simulink library "inp"  (R2021b)
settings: Solver=VariableStepAuto  StartTime=0.0  StopTime=10.0  RelTol=1e-3
undefined symbols (not defined in the file): C_TASK_5MS_S, FALSE, KINP_AcoreReadyToSlp_flg_ovrdflg, KINP_AcoreReadyToSlp_flg_ovrdval, KINP_AllowMovThd_OTA_enum_ovrdflg, KINP_AllowMovThd_OTA_enum_ovrdval, KINP_APSAngleTarget_Deg_ovrdflg, KINP_APSAngleTarget_Deg_ovrdval, KINP_APSDecReq_mps2_ovrdflg, KINP_APSDecReq_mps2_ovrdval, KINP_APSDecReqA_flg_ovrdflg, KINP_APSDecReqA_flg_ovrdval, KINP_APSDFLL_cm_ovrdflg, KINP_APSDFLL_cm_ovrdval, KINP_APSDFLR_cm_ovrdflg, KINP_APSDFLR_cm_ovrdval, KINP_APSDRLL_cm_ovrdflg, KINP_APSDRLL_cm_ovrdval, KINP_APSDRLR_cm_ovrdflg, KINP_APSDRLR_cm_ovrdval, KINP_APSExitCondition_enum_ovrdflg, KINP_APSExitCondition_enum_ovrdval, KINP_APSHWVer_enum_ovrdflg, KINP_APSHWVer_enum_ovrdval, KINP_APSProgressPCT_pct_ovrdflg, KINP_APSProgressPCT_pct_ovrdval, KINP_APSReq_enum_ovrdflg, KINP_APSReq_enum_ovrdval, KINP_APSRQDisplay_enum_ovrdflg, KINP_APSRQDisplay_enum_ovrdval, KINP_APSRqEPASCtrl_flg_ovrdflg, KINP_APSRqEPASCtrl_flg_ovrdval, KINP_APSShiftPosnReq_enum_ovrdval, KINP_APSShiftPosnReq_enum_ovrflg, KINP_APSSpeedCMD_kph_ovrdval, KINP_APSSpeedCMD_kph_ovrflg, KINP_APSStaSystem_enum_ovrdflg, KINP_APSStaSystem_enum_ovrdval, KINP_APSSWVer_enum_ovrdflg, KINP_APSSWVer_enum_ovrdval, KINP_APSVMCReqA_flg_ovrdval, KINP_APSVMCReqA_flg_ovrflg, KINP_APSVRqEPASCtrl_flg_ovrdflg, KINP_APSVRqEPASCtrl_flg_ovrdval, KINP_AuxBattVolmV_mV_ovrdflg, KINP_AuxBattVolmV_mV_ovrdval, KINP_CAASSta_enum_ovrdflg, KINP_CAASSta_enum_ovrdval, KINP_CAASVMCReqA_flg_ovrdval, KINP_CAASVMCReqA_flg_ovrflg, KINP_Chime_enum_ovrdflg, KINP_Chime_enum_ovrdval, KINP_ClearDTCcmd_flg_ovrdflg, KINP_ClearDTCcmd_flg_ovrdval, KINP_EvccAplusPwrUpReq_flg_ovrdflg, KINP_EvccAplusPwrUpReq_flg_ovrdval, KINP_LFID_raw_ovrdval, KINP_LFID_raw_ovrflg, KINP_LRID_raw_ovrdval, KINP_MemOffsetAccX_raw16_ovrdflg ... (+118)
libraries: FVT_lib x595, hcu_lib x1
(part 12 of 27)

== system inp/INP/CAN1/SignalCheck/FCM3 ==
  BHAL_outputs : Inport
  inp_CanValid_bus : Inport  Port=2
  ACCObjDist : FVT_lib/inp/can_signal_template  SystemSampleTime=-1  VariantActivationTime=update diagram  Latency=0  AutoFrameSizeCalculation=off
      link override defval: Value=KINP_ACCObjDist_m_defval
      link override fftdec: Value=KINP_ACCObjDist_m_fftdec
      link override fftinc: Value=KINP_ACCObjDist_m_fftinc
      link override fftlim: Value=KINP_ACCObjDist_m_fftlim
      link override invalid: Value=KINP_ACCObjDist_m_invalid
      link override ovrdflg: Value=KINP_ACCObjDist_m_ovrdflg
      link override ovrdval: Value=KINP_ACCObjDist_m_ovrdval
      link override setvalid: Value=KINP_ACCObjDist_m_setvalid
      link override srvcflg: Value=KINP_ACCObjDist_m_srvcflg
      link override srvcval: Value=KINP_ACCObjDist_m_srvcval
  ACCObjRelSpd : FVT_lib/inp/can_signal_template  SystemSampleTime=-1  VariantActivationTime=update diagram  Latency=0  AutoFrameSizeCalculation=off
      link override defval: Value=KINP_ACCObjRelSpd_mps_defval
      link override fftdec: Value=KINP_ACCObjRelSpd_mps_fftdec
      link override fftinc: Value=KINP_ACCObjRelSpd_mps_fftinc
      link override fftlim: Value=KINP_ACCObjRelSpd_mps_fftlim
      link override invalid: Value=KINP_ACCObjRelSpd_mps_invalid
      link override ovrdflg: Value=KINP_ACCObjRelSpd_mps_ovrdflg
      link override ovrdval: Value=KINP_ACCObjRelSpd_mps_ovrdval
      link override setvalid: Value=KINP_ACCObjRelSpd_mps_setvalid
      link override srvcflg: Value=KINP_ACCObjRelSpd_mps_srvcflg
      link override srvcval: Value=KINP_ACCObjRelSpd_mps_srvcval
  ADASForceIdle : FVT_lib/inp/can_signal_template  SystemSampleTime=-1  VariantActivationTime=update diagram  Latency=0  AutoFrameSizeCalculation=off
      link override defval: Value=KINP_ADASForceIdle_flg_defval
      link override fftdec: Value=KINP_ADASForceIdle_flg_fftdec
      link override fftinc: Value=KINP_ADASForceIdle_flg_fftinc
      link override fftlim: Value=KINP_ADASForceIdle_flg_fftlim
      link override invalid: Value=KINP_ADASForceIdle_flg_invalid
      link override ovrdflg: Value=KINP_ADASForceIdle_flg_ovrdflg
      link override ovrdval: Value=KINP_ADASForceIdle_flg_ovrdval
      link override setvalid: Value=KINP_ADASForceIdle_flg_setvalid
      link override srvcflg: Value=KINP_ADASForceIdle_flg_srvcflg
      link override srvcval: Value=KINP_ADASForceIdle_flg_srvcval
  FCM3CSErr : FVT_lib/inp/can_signal_template  SystemSampleTime=-1  VariantActivationTime=update diagram  Latency=0  AutoFrameSizeCalculation=off
      link override defval: Value=KINP_FCM3CSErr_flg_defval
      link override fftdec: Value=KINP_FCM3CSErr_flg_fftdec
      link override fftinc: Value=KINP_FCM3CSErr_flg_fftinc
      link override fftlim: Value=KINP_FCM3CSErr_flg_fftlim
      link override invalid: Value=KINP_FCM3CSErr_flg_invalid
      link override ovrdflg: Value=KINP_FCM3CSErr_flg_ovrdflg
      link override ovrdval: Value=KINP_FCM3CSErr_flg_ovrdval
      link override setvalid: Value=KINP_FCM3CSErr_flg_setvalid
      link override srvcflg: Value=KINP_FCM3CSErr_flg_srvcflg
      link override srvcval: Value=KINP_FCM3CSErr_flg_srvcval
  FCM3Checksum : FVT_lib/inp/can_signal_template  SystemSampleTime=-1  VariantActivationTime=update diagram  Latency=0  AutoFrameSizeCalculation=off
      link override defval: Value=KINP_FCM3Checksum_enum_defval
      link override fftdec: Value=KINP_FCM3Checksum_enum_fftdec
      link override fftinc: Value=KINP_FCM3Checksum_enum_fftinc
      link override fftlim: Value=KINP_FCM3Checksum_enum_fftlim
      link override invalid: Value=KINP_FCM3Checksum_enum_invalid
      link override ovrdflg: Value=KINP_FCM3Checksum_enum_ovrdflg
      link override ovrdval: Value=KINP_FCM3Checksum_enum_ovrdval
      link override setvalid: Value=KINP_FCM3Checksum_enum_setvalid
      link override srvcflg: Value=KINP_FCM3Checksum_enum_srvcflg
      link override srvcval: Value=KINP_FCM3Checksum_enum_srvcval
  FCM3LifeCount : FVT_lib/inp/can_signal_template  SystemSampleTime=-1  VariantActivationTime=update diagram  Latency=0  AutoFrameSizeCalculation=off
      link override defval: Value=KINP_FCM3LifeCount_enum_defval
      link override fftdec: Value=KINP_FCM3LifeCount_enum_fftdec
      link override fftinc: Value=KINP_FCM3LifeCount_enum_fftinc
      link override fftlim: Value=KINP_FCM3LifeCount_enum_fftlim
      link override invalid: Value=KINP_FCM3LifeCount_enum_invalid
      link override ovrdflg: Value=KINP_FCM3LifeCount_enum_ovrdflg
      link override ovrdval: Value=KINP_FCM3LifeCount_enum_ovrdval
      link override setvalid: Value=KINP_FCM3LifeCount_enum_setvalid
      link override srvcflg: Value=KINP_FCM3LifeCount_enum_srvcflg
      link override srvcval: Value=KINP_FCM3LifeCount_enum_srvcval
  FCM3RCErr : FVT_lib/inp/can_signal_template  SystemSampleTime=-1  VariantActivationTime=update diagram  Latency=0  AutoFrameSizeCalculation=off
      link override defval: Value=KINP_FCM3RCErr_flg_defval
      link override fftdec: Value=KINP_FCM3RCErr_flg_fftdec
      link override fftinc: Value=KINP_FCM3RCErr_flg_fftinc
      link override fftlim: Value=KINP_FCM3RCErr_flg_fftlim
      link override invalid: Value=KINP_FCM3RCErr_flg_invalid
      link override ovrdflg: Value=KINP_FCM3RCErr_flg_ovrdflg
      link override ovrdval: Value=KINP_FCM3RCErr_flg_ovrdval
      link override setvalid: Value=KINP_FCM3RCErr_flg_setvalid
      link override srvcflg: Value=KINP_FCM3RCErr_flg_srvcflg
      link override srvcval: Value=KINP_FCM3RCErr_flg_srvcval
  Terminator_{1..7} (7 alike) : Terminator
  True_VHAL_ACCObjDist_m : Constant  Value=TRUE  OutDataTypeStr=boolean
  True_VHAL_ACCObjRelSpd_mps : Constant  Value=TRUE  OutDataTypeStr=boolean
  True_VHAL_ADASForceIdle_flg : Constant  Value=TRUE  OutDataTypeStr=boolean
  True_VHAL_FCM3CSErr_flg : Constant  Value=TRUE  OutDataTypeStr=boolean
  True_VHAL_FCM3Checksum_enum : Constant  Value=TRUE  OutDataTypeStr=boolean
  True_VHAL_FCM3LifeCount_enum : Constant  Value=TRUE  OutDataTypeStr=boolean
  True_VHAL_FCM3RCErr_flg : Constant  Value=TRUE  OutDataTypeStr=boolean
  slr1_{1..7} (7 alike) : BusSelector  OutputSignals=VINP_CANMsgValidFCM3_flg
  slr_VHAL_ACCObjDist_m : BusSelector  OutputSignals=VHAL_ACCObjDist_m
  slr_VHAL_ACCObjRelSpd_mps : BusSelector  OutputSignals=VHAL_ACCObjRelSpd_mps
  slr_VHAL_ADASForceIdle_flg : BusSelector  OutputSignals=VHAL_ADASForceIdle_flg
  slr_VHAL_FCM3CSErr_flg : BusSelector  OutputSignals=VHAL_FCM3CSErr_flg
  slr_VHAL_FCM3Checksum_enum : BusSelector  OutputSignals=VHAL_FCM3Checksum_enum
  slr_VHAL_FCM3LifeCount_enum : BusSelector  OutputSignals=VHAL_FCM3LifeCount_enum
  slr_VHAL_FCM3RCErr_flg : BusSelector  OutputSignals=VHAL_FCM3RCErr_flg
  VINP_FCM3CSErr_flg : Outport
  VINP_FCM3RCErr_flg : Outport  Port=2
  VINP_ACCObjDist_m : Outport  Port=3
  VINP_ACCObjRelSpd_mps : Outport  Port=4
  VINP_ADASForceIdle_flg : Outport  Port=5
  VINP_FCM3Checksum_enum : Outport  Port=6
  VINP_FCM3LifeCount_enum : Outport  Port=7
  wires:
  BHAL_outputs/1 -> [BHAL_outputs]
  inp_CanValid_bus/1 -> [inp_CanValid_bus]
  [BHAL_outputs] -> slr_VHAL_FCM3CSErr_flg/1
  slr_VHAL_FCM3CSErr_flg/1 -> FCM3CSErr/1  "<VHAL_FCM3CSErr_flg>"
  True_VHAL_FCM3CSErr_flg/1 -> FCM3CSErr/2
  [inp_CanValid_bus] -> slr1_1/1
  slr1_1/1 -> FCM3CSErr/3  "<VINP_CANMsgValidFCM3_flg>"
  FCM3CSErr/1 -> VINP_FCM3CSErr_flg/1  "VINP_FCM3CSErr_flg"
  FCM3CSErr/2 -> Terminator_1/1
  [BHAL_outputs] -> slr_VHAL_FCM3RCErr_flg/1
  slr_VHAL_FCM3RCErr_flg/1 -> FCM3RCErr/1  "<VHAL_FCM3RCErr_flg>"
  True_VHAL_FCM3RCErr_flg/1 -> FCM3RCErr/2
  [inp_CanValid_bus] -> slr1_2/1
  slr1_2/1 -> FCM3RCErr/3  "<VINP_CANMsgValidFCM3_flg>"
  FCM3RCErr/1 -> VINP_FCM3RCErr_flg/1  "VINP_FCM3RCErr_flg"
  FCM3RCErr/2 -> Terminator_2/1
  [BHAL_outputs] -> slr_VHAL_ACCObjDist_m/1
  slr_VHAL_ACCObjDist_m/1 -> ACCObjDist/1  "<VHAL_ACCObjDist_m>"
  True_VHAL_ACCObjDist_m/1 -> ACCObjDist/2
  [inp_CanValid_bus] -> slr1_3/1
  slr1_3/1 -> ACCObjDist/3  "<VINP_CANMsgValidFCM3_flg>"
  ACCObjDist/1 -> VINP_ACCObjDist_m/1  "VINP_ACCObjDist_m"
  ACCObjDist/2 -> Terminator_3/1
  [BHAL_outputs] -> slr_VHAL_ACCObjRelSpd_mps/1
  slr_VHAL_ACCObjRelSpd_mps/1 -> ACCObjRelSpd/1  "<VHAL_ACCObjRelSpd_mps>"
  True_VHAL_ACCObjRelSpd_mps/1 -> ACCObjRelSpd/2
  [inp_CanValid_bus] -> slr1_4/1
  slr1_4/1 -> ACCObjRelSpd/3  "<VINP_CANMsgValidFCM3_flg>"
  ACCObjRelSpd/1 -> VINP_ACCObjRelSpd_mps/1  "VINP_ACCObjRelSpd_mps"
  ACCObjRelSpd/2 -> Terminator_4/1
  [BHAL_outputs] -> slr_VHAL_ADASForceIdle_flg/1
  slr_VHAL_ADASForceIdle_flg/1 -> ADASForceIdle/1  "<VHAL_ADASForceIdle_flg>"
  True_VHAL_ADASForceIdle_flg/1 -> ADASForceIdle/2
  [inp_CanValid_bus] -> slr1_5/1
  slr1_5/1 -> ADASForceIdle/3  "<VINP_CANMsgValidFCM3_flg>"
  ADASForceIdle/1 -> VINP_ADASForceIdle_flg/1  "VINP_ADASForceIdle_flg"
  ADASForceIdle/2 -> Terminator_5/1
  [BHAL_outputs] -> slr_VHAL_FCM3Checksum_enum/1
  slr_VHAL_FCM3Checksum_enum/1 -> FCM3Checksum/1  "<VHAL_FCM3Checksum_enum>"
  True_VHAL_FCM3Checksum_enum/1 -> FCM3Checksum/2
  [inp_CanValid_bus] -> slr1_6/1
  slr1_6/1 -> FCM3Checksum/3  "<VINP_CANMsgValidFCM3_flg>"
  FCM3Checksum/1 -> VINP_FCM3Checksum_enum/1  "VINP_FCM3Checksum_enum"
  FCM3Checksum/2 -> Terminator_6/1
  [BHAL_outputs] -> slr_VHAL_FCM3LifeCount_enum/1
  slr_VHAL_FCM3LifeCount_enum/1 -> FCM3LifeCount/1  "<VHAL_FCM3LifeCount_enum>"
  True_VHAL_FCM3LifeCount_enum/1 -> FCM3LifeCount/2
  [inp_CanValid_bus] -> slr1_7/1
  slr1_7/1 -> FCM3LifeCount/3  "<VINP_CANMsgValidFCM3_flg>"
  FCM3LifeCount/1 -> VINP_FCM3LifeCount_enum/1  "VINP_FCM3LifeCount_enum"
  FCM3LifeCount/2 -> Terminator_7/1

== system inp/INP/CAN1/SignalCheck/FCM4 ==
  BHAL_outputs : Inport
  inp_CanValid_bus : Inport  Port=2
  ACCSetSpeed : FVT_lib/inp/can_signal_template  SystemSampleTime=-1  VariantActivationTime=update diagram  Latency=0  AutoFrameSizeCalculation=off
      link override defval: Value=KINP_ACCSetSpeed_enum_defval
      link override fftdec: Value=KINP_ACCSetSpeed_enum_fftdec
      link override fftinc: Value=KINP_ACCSetSpeed_enum_fftinc
      link override fftlim: Value=KINP_ACCSetSpeed_enum_fftlim
      link override invalid: Value=KINP_ACCSetSpeed_enum_invalid
      link override ovrdflg: Value=KINP_ACCSetSpeed_enum_ovrdflg
      link override ovrdval: Value=KINP_ACCSetSpeed_enum_ovrdval
      link override setvalid: Value=KINP_ACCSetSpeed_enum_setvalid
      link override srvcflg: Value=KINP_ACCSetSpeed_enum_srvcflg
      link override srvcval: Value=KINP_ACCSetSpeed_enum_srvcval
  ACCSetSpeedDisp : FVT_lib/inp/can_signal_template  SystemSampleTime=-1  VariantActivationTime=update diagram  Latency=0  AutoFrameSizeCalculation=off
      link override defval: Value=KINP_ACCSetSpeedDisp_enum_defval
      link override fftdec: Value=KINP_ACCSetSpeedDisp_enum_fftdec
      link override fftinc: Value=KINP_ACCSetSpeedDisp_enum_fftinc
      link override fftlim: Value=KINP_ACCSetSpeedDisp_enum_fftlim
      link override invalid: Value=KINP_ACCSetSpeedDisp_enum_invalid
      link override ovrdflg: Value=KINP_ACCSetSpeedDisp_enum_ovrdflg
      link override ovrdval: Value=KINP_ACCSetSpeedDisp_enum_ovrdval
      link override setvalid: Value=KINP_ACCSetSpeedDisp_enum_setvalid
      link override srvcflg: Value=KINP_ACCSetSpeedDisp_enum_srvcflg
      link override srvcval: Value=KINP_ACCSetSpeedDisp_enum_srvcval
  ADASACCSta : FVT_lib/inp/can_signal_template  SystemSampleTime=-1  VariantActivationTime=update diagram  Latency=0  AutoFrameSizeCalculation=off
      link override defval: Value=KINP_ADASACCSta_enum_defval
      link override fftdec: Value=KINP_ADASACCSta_enum_fftdec
      link override fftinc: Value=KINP_ADASACCSta_enum_fftinc
      link override fftlim: Value=KINP_ADASACCSta_enum_fftlim
      link override invalid: Value=KINP_ADASACCSta_enum_invalid
      link override ovrdflg: Value=KINP_ADASACCSta_enum_ovrdflg
      link override ovrdval: Value=KINP_ADASACCSta_enum_ovrdval
      link override setvalid: Value=KINP_ADASACCSta_enum_setvalid
      link override srvcflg: Value=KINP_ADASACCSta_enum_srvcflg
      link override srvcval: Value=KINP_ADASACCSta_enum_srvcval
  FCM4CSErr : FVT_lib/inp/can_signal_template  SystemSampleTime=-1  VariantActivationTime=update diagram  Latency=0  AutoFrameSizeCalculation=off
      link override defval: Value=KINP_FCM4CSErr_flg_defval
      link override fftdec: Value=KINP_FCM4CSErr_flg_fftdec
      link override fftinc: Value=KINP_FCM4CSErr_flg_fftinc
      link override fftlim: Value=KINP_FCM4CSErr_flg_fftlim
      link override invalid: Value=KINP_FCM4CSErr_flg_invalid
      link override ovrdflg: Value=KINP_FCM4CSErr_flg_ovrdflg
      link override ovrdval: Value=KINP_FCM4CSErr_flg_ovrdval
      link override setvalid: Value=KINP_FCM4CSErr_flg_setvalid
      link override srvcflg: Value=KINP_FCM4CSErr_flg_srvcflg
      link override srvcval: Value=KINP_FCM4CSErr_flg_srvcval
  FCM4Checksum : FVT_lib/inp/can_signal_template  SystemSampleTime=-1  VariantActivationTime=update diagram  Latency=0  AutoFrameSizeCalculation=off
      link override defval: Value=KINP_FCM4Checksum_enum_defval
      link override fftdec: Value=KINP_FCM4Checksum_enum_fftdec
      link override fftinc: Value=KINP_FCM4Checksum_enum_fftinc
      link override fftlim: Value=KINP_FCM4Checksum_enum_fftlim
      link override invalid: Value=KINP_FCM4Checksum_enum_invalid
      link override ovrdflg: Value=KINP_FCM4Checksum_enum_ovrdflg
      link override ovrdval: Value=KINP_FCM4Checksum_enum_ovrdval
      link override setvalid: Value=KINP_FCM4Checksum_enum_setvalid
      link override srvcflg: Value=KINP_FCM4Checksum_enum_srvcflg
      link override srvcval: Value=KINP_FCM4Checksum_enum_srvcval
  FCM4RCErr : FVT_lib/inp/can_signal_template  SystemSampleTime=-1  VariantActivationTime=update diagram  Latency=0  AutoFrameSizeCalculation=off
      link override defval: Value=KINP_FCM4RCErr_flg_defval
      link override fftdec: Value=KINP_FCM4RCErr_flg_fftdec
      link override fftinc: Value=KINP_FCM4RCErr_flg_fftinc
      link override fftlim: Value=KINP_FCM4RCErr_flg_fftlim
      link override invalid: Value=KINP_FCM4RCErr_flg_invalid
      link override ovrdflg: Value=KINP_FCM4RCErr_flg_ovrdflg
      link override ovrdval: Value=KINP_FCM4RCErr_flg_ovrdval
      link override setvalid: Value=KINP_FCM4RCErr_flg_setvalid
      link override srvcflg: Value=KINP_FCM4RCErr_flg_srvcflg
      link override srvcval: Value=KINP_FCM4RCErr_flg_srvcval
  ForceLowBeam : FVT_lib/inp/can_signal_template  SystemSampleTime=-1  VariantActivationTime=update diagram  Latency=0  AutoFrameSizeCalculation=off
      link override defval: Value=KINP_ForceLowBeam_enum_defval
      link override fftdec: Value=KINP_ForceLowBeam_enum_fftdec
      link override fftinc: Value=KINP_ForceLowBeam_enum_fftinc
      link override fftlim: Value=KINP_ForceLowBeam_enum_fftlim
      link override invalid: Value=KINP_ForceLowBeam_enum_invalid
      link override ovrdflg: Value=KINP_ForceLowBeam_enum_ovrdflg
      link override ovrdval: Value=KINP_ForceLowBeam_enum_ovrdval
      link override setvalid: Value=KINP_ForceLowBeam_enum_setvalid
      link override srvcflg: Value=KINP_ForceLowBeam_enum_srvcflg
      link override srvcval: Value=KINP_ForceLowBeam_enum_srvcval
  HazardWarningReq : FVT_lib/inp/can_signal_template  SystemSampleTime=-1  VariantActivationTime=update diagram  Latency=0  AutoFrameSizeCalculation=off
      link override defval: Value=KINP_HazardWarningReq_flg_defval
      link override fftdec: Value=KINP_HazardWarningReq_flg_fftdec
      link override fftinc: Value=KINP_HazardWarningReq_flg_fftinc
      link override fftlim: Value=KINP_HazardWarningReq_flg_fftlim
      link override invalid: Value=KINP_HazardWarningReq_flg_invalid
      link override ovrdflg: Value=KINP_HazardWarningReq_flg_ovrdflg
      link override ovrdval: Value=KINP_HazardWarningReq_flg_ovrdval
      link override setvalid: Value=KINP_HazardWarningReq_flg_setvalid
      link override srvcflg: Value=KINP_HazardWarningReq_flg_srvcflg
      link override srvcval: Value=KINP_HazardWarningReq_flg_srvcval
  LeftTurnLightReq : FVT_lib/inp/can_signal_template  SystemSampleTime=-1  VariantActivationTime=update diagram  Latency=0  AutoFrameSizeCalculation=off
      link override defval: Value=KINP_LeftTurnLightReq_flg_defval
      link override fftdec: Value=KINP_LeftTurnLightReq_flg_fftdec
      link override fftinc: Value=KINP_LeftTurnLightReq_flg_fftinc
      link override fftlim: Value=KINP_LeftTurnLightReq_flg_fftlim
      link override invalid: Value=KINP_LeftTurnLightReq_flg_invalid
      link override ovrdflg: Value=KINP_LeftTurnLightReq_flg_ovrdflg
      link override ovrdval: Value=KINP_LeftTurnLightReq_flg_ovrdval
      link override setvalid: Value=KINP_LeftTurnLightReq_flg_setvalid
      link override srvcflg: Value=KINP_LeftTurnLightReq_flg_srvcflg
      link override srvcval: Value=KINP_LeftTurnLightReq_flg_srvcval
  RightTurnLightReq : FVT_lib/inp/can_signal_template  SystemSampleTime=-1  VariantActivationTime=update diagram  Latency=0  AutoFrameSizeCalculation=off
      link override defval: Value=KINP_RightTurnLightReq_flg_defval
      link override fftdec: Value=KINP_RightTurnLightReq_flg_fftdec
      link override fftinc: Value=KINP_RightTurnLightReq_flg_fftinc
      link override fftlim: Value=KINP_RightTurnLightReq_flg_fftlim
      link override invalid: Value=KINP_RightTurnLightReq_flg_invalid
      link override ovrdflg: Value=KINP_RightTurnLightReq_flg_ovrdflg
      link override ovrdval: Value=KINP_RightTurnLightReq_flg_ovrdval
      link override setvalid: Value=KINP_RightTurnLightReq_flg_setvalid
      link override srvcflg: Value=KINP_RightTurnLightReq_flg_srvcflg
      link override srvcval: Value=KINP_RightTurnLightReq_flg_srvcval
  TargetType : FVT_lib/inp/can_signal_template  SystemSampleTime=-1  VariantActivationTime=update diagram  Latency=0  AutoFrameSizeCalculation=off
      link override defval: Value=KINP_TargetType_enum_defval
      link override fftdec: Value=KINP_TargetType_enum_fftdec
      link override fftinc: Value=KINP_TargetType_enum_fftinc
      link override fftlim: Value=KINP_TargetType_enum_fftlim
      link override invalid: Value=KINP_TargetType_enum_invalid
      link override ovrdflg: Value=KINP_TargetType_enum_ovrdflg
      link override ovrdval: Value=KINP_TargetType_enum_ovrdval
      link override setvalid: Value=KINP_TargetType_enum_setvalid
      link override srvcflg: Value=KINP_TargetType_enum_srvcflg
      link override srvcval: Value=KINP_TargetType_enum_srvcval
  Terminator_{1..12} (12 alike) : Terminator
  TimeGapLevel : FVT_lib/inp/can_signal_template  SystemSampleTime=-1  VariantActivationTime=update diagram  Latency=0  AutoFrameSizeCalculation=off
      link override defval: Value=KINP_TimeGapLevel_enum_defval
      link override fftdec: Value=KINP_TimeGapLevel_enum_fftdec
      link override fftinc: Value=KINP_TimeGapLevel_enum_fftinc
      link override fftlim: Value=KINP_TimeGapLevel_enum_fftlim
      link override invalid: Value=KINP_TimeGapLevel_enum_invalid
      link override ovrdflg: Value=KINP_TimeGapLevel_enum_ovrdflg
      link override ovrdval: Value=KINP_TimeGapLevel_enum_ovrdval
      link override setvalid: Value=KINP_TimeGapLevel_enum_setvalid
      link override srvcflg: Value=KINP_TimeGapLevel_enum_srvcflg
      link override srvcval: Value=KINP_TimeGapLevel_enum_srvcval
  True_VHAL_ACCSetSpeedDisp_enum : Constant  Value=TRUE  OutDataTypeStr=boolean
  True_VHAL_ACCSetSpeed_enum : Constant  Value=TRUE  OutDataTypeStr=boolean
  True_VHAL_ADASACCSta_enum : Constant  Value=TRUE  OutDataTypeStr=boolean
  True_VHAL_FCM4CSErr_flg : Constant  Value=TRUE  OutDataTypeStr=boolean
  True_VHAL_FCM4Checksum_enum : Constant  Value=TRUE  OutDataTypeStr=boolean
  True_VHAL_FCM4RCErr_flg : Constant  Value=TRUE  OutDataTypeStr=boolean
  True_VHAL_ForceLowBeam_enum : Constant  Value=TRUE  OutDataTypeStr=boolean
  True_VHAL_HazardWarningReq_flg : Constant  Value=TRUE  OutDataTypeStr=boolean
  True_VHAL_LeftTurnLightReq_flg : Constant  Value=TRUE  OutDataTypeStr=boolean
  True_VHAL_RightTurnLightReq_flg : Constant  Value=TRUE  OutDataTypeStr=boolean
  True_VHAL_TargetType_enum : Constant  Value=TRUE  OutDataTypeStr=boolean
  True_VHAL_TimeGapLevel_enum : Constant  Value=TRUE  OutDataTypeStr=boolean
  slr1_{1..12} (12 alike) : BusSelector  OutputSignals=VINP_CANMsgValidFCM4_flg
  slr_VHAL_ACCSetSpeedDisp_enum : BusSelector  OutputSignals=VHAL_ACCSetSpeedDisp_enum
  slr_VHAL_ACCSetSpeed_enum : BusSelector  OutputSignals=VHAL_ACCSetSpeed_enum
  slr_VHAL_ADASACCSta_enum : BusSelector  OutputSignals=VHAL_ADASACCSta_enum
  slr_VHAL_FCM4CSErr_flg : BusSelector  OutputSignals=VHAL_FCM4CSErr_flg
  slr_VHAL_FCM4Checksum_enum : BusSelector  OutputSignals=VHAL_FCM4Checksum_enum
  slr_VHAL_FCM4RCErr_flg : BusSelector  OutputSignals=VHAL_FCM4RCErr_flg
  slr_VHAL_ForceLowBeam_enum : BusSelector  OutputSignals=VHAL_ForceLowBeam_enum
  slr_VHAL_HazardWarningReq_flg : BusSelector  OutputSignals=VHAL_HazardWarningReq_flg
  slr_VHAL_LeftTurnLightReq_flg : BusSelector  OutputSignals=VHAL_LeftTurnLightReq_flg
  slr_VHAL_RightTurnLightReq_flg : BusSelector  OutputSignals=VHAL_RightTurnLightReq_flg
  slr_VHAL_TargetType_enum : BusSelector  OutputSignals=VHAL_TargetType_enum
  slr_VHAL_TimeGapLevel_enum : BusSelector  OutputSignals=VHAL_TimeGapLevel_enum
  VINP_FCM4CSErr_flg : Outport
  VINP_FCM4RCErr_flg : Outport  Port=2
  VINP_ACCSetSpeed_enum : Outport  Port=3
  VINP_ACCSetSpeedDisp_enum : Outport  Port=4
  VINP_ADASACCSta_enum : Outport  Port=5
  VINP_FCM4Checksum_enum : Outport  Port=6
  VINP_ForceLowBeam_enum : Outport  Port=7
  VINP_HazardWarningReq_flg : Outport  Port=8
  VINP_LeftTurnLightReq_flg : Outport  Port=9
  VINP_RightTurnLightReq_flg : Outport  Port=10
  VINP_TargetType_enum : Outport  Port=11
  VINP_TimeGapLevel_enum : Outport  Port=12
  wires:
  BHAL_outputs/1 -> [BHAL_outputs]
  inp_CanValid_bus/1 -> [inp_CanValid_bus]
  [BHAL_outputs] -> slr_VHAL_FCM4CSErr_flg/1
  slr_VHAL_FCM4CSErr_flg/1 -> FCM4CSErr/1  "<VHAL_FCM4CSErr_flg>"
  True_VHAL_FCM4CSErr_flg/1 -> FCM4CSErr/2
  [inp_CanValid_bus] -> slr1_1/1
  slr1_1/1 -> FCM4CSErr/3  "<VINP_CANMsgValidFCM4_flg>"
  FCM4CSErr/1 -> VINP_FCM4CSErr_flg/1  "VINP_FCM4CSErr_flg"
  FCM4CSErr/2 -> Terminator_1/1
  [BHAL_outputs] -> slr_VHAL_FCM4RCErr_flg/1
  slr_VHAL_FCM4RCErr_flg/1 -> FCM4RCErr/1  "<VHAL_FCM4RCErr_flg>"
  True_VHAL_FCM4RCErr_flg/1 -> FCM4RCErr/2
  [inp_CanValid_bus] -> slr1_2/1
  slr1_2/1 -> FCM4RCErr/3  "<VINP_CANMsgValidFCM4_flg>"
  FCM4RCErr/1 -> VINP_FCM4RCErr_flg/1  "VINP_FCM4RCErr_flg"
  FCM4RCErr/2 -> Terminator_2/1
  [BHAL_outputs] -> slr_VHAL_ACCSetSpeed_enum/1
  slr_VHAL_ACCSetSpeed_enum/1 -> ACCSetSpeed/1  "<VHAL_ACCSetSpeed_enum>"
  True_VHAL_ACCSetSpeed_enum/1 -> ACCSetSpeed/2
  [inp_CanValid_bus] -> slr1_3/1
  slr1_3/1 -> ACCSetSpeed/3  "<VINP_CANMsgValidFCM4_flg>"
  ACCSetSpeed/1 -> VINP_ACCSetSpeed_enum/1  "VINP_ACCSetSpeed_enum"
  ACCSetSpeed/2 -> Terminator_3/1
  [BHAL_outputs] -> slr_VHAL_ACCSetSpeedDisp_enum/1
  slr_VHAL_ACCSetSpeedDisp_enum/1 -> ACCSetSpeedDisp/1  "<VHAL_ACCSetSpeedDisp_enum>"
  True_VHAL_ACCSetSpeedDisp_enum/1 -> ACCSetSpeedDisp/2
  [inp_CanValid_bus] -> slr1_4/1
  slr1_4/1 -> ACCSetSpeedDisp/3  "<VINP_CANMsgValidFCM4_flg>"
  ACCSetSpeedDisp/1 -> VINP_ACCSetSpeedDisp_enum/1  "VINP_ACCSetSpeedDisp_enum"
  ACCSetSpeedDisp/2 -> Terminator_4/1
  [BHAL_outputs] -> slr_VHAL_ADASACCSta_enum/1
  slr_VHAL_ADASACCSta_enum/1 -> ADASACCSta/1  "<VHAL_ADASACCSta_enum>"
  True_VHAL_ADASACCSta_enum/1 -> ADASACCSta/2
  [inp_CanValid_bus] -> slr1_5/1
  slr1_5/1 -> ADASACCSta/3  "<VINP_CANMsgValidFCM4_flg>"
  ADASACCSta/1 -> VINP_ADASACCSta_enum/1  "VINP_ADASACCSta_enum"
  ADASACCSta/2 -> Terminator_5/1
  [BHAL_outputs] -> slr_VHAL_FCM4Checksum_enum/1
  slr_VHAL_FCM4Checksum_enum/1 -> FCM4Checksum/1  "<VHAL_FCM4Checksum_enum>"
  True_VHAL_FCM4Checksum_enum/1 -> FCM4Checksum/2
  [inp_CanValid_bus] -> slr1_6/1
  slr1_6/1 -> FCM4Checksum/3  "<VINP_CANMsgValidFCM4_flg>"
  FCM4Checksum/1 -> VINP_FCM4Checksum_enum/1  "VINP_FCM4Checksum_enum"
  FCM4Checksum/2 -> Terminator_6/1
  [BHAL_outputs] -> slr_VHAL_ForceLowBeam_enum/1
  slr_VHAL_ForceLowBeam_enum/1 -> ForceLowBeam/1  "<VHAL_ForceLowBeam_enum>"
  True_VHAL_ForceLowBeam_enum/1 -> ForceLowBeam/2
  [inp_CanValid_bus] -> slr1_7/1
  slr1_7/1 -> ForceLowBeam/3  "<VINP_CANMsgValidFCM4_flg>"
  ForceLowBeam/1 -> VINP_ForceLowBeam_enum/1  "VINP_ForceLowBeam_enum"
  ForceLowBeam/2 -> Terminator_7/1
  [BHAL_outputs] -> slr_VHAL_HazardWarningReq_flg/1
  slr_VHAL_HazardWarningReq_flg/1 -> HazardWarningReq/1  "<VHAL_HazardWarningReq_flg>"
  True_VHAL_HazardWarningReq_flg/1 -> HazardWarningReq/2
  [inp_CanValid_bus] -> slr1_8/1
  slr1_8/1 -> HazardWarningReq/3  "<VINP_CANMsgValidFCM4_flg>"
  HazardWarningReq/1 -> VINP_HazardWarningReq_flg/1  "VINP_HazardWarningReq_flg"
  HazardWarningReq/2 -> Terminator_8/1
  [BHAL_outputs] -> slr_VHAL_LeftTurnLightReq_flg/1
  slr_VHAL_LeftTurnLightReq_flg/1 -> LeftTurnLightReq/1  "<VHAL_LeftTurnLightReq_flg>"
  True_VHAL_LeftTurnLightReq_flg/1 -> LeftTurnLightReq/2
  [inp_CanValid_bus] -> slr1_9/1
  slr1_9/1 -> LeftTurnLightReq/3  "<VINP_CANMsgValidFCM4_flg>"
  LeftTurnLightReq/1 -> VINP_LeftTurnLightReq_flg/1  "VINP_LeftTurnLightReq_flg"
  LeftTurnLightReq/2 -> Terminator_9/1
  [BHAL_outputs] -> slr_VHAL_RightTurnLightReq_flg/1
  slr_VHAL_RightTurnLightReq_flg/1 -> RightTurnLightReq/1  "<VHAL_RightTurnLightReq_flg>"
  True_VHAL_RightTurnLightReq_flg/1 -> RightTurnLightReq/2
  [inp_CanValid_bus] -> slr1_10/1
  slr1_10/1 -> RightTurnLightReq/3  "<VINP_CANMsgValidFCM4_flg>"
  RightTurnLightReq/1 -> VINP_RightTurnLightReq_flg/1  "VINP_RightTurnLightReq_flg"
  RightTurnLightReq/2 -> Terminator_10/1
  [BHAL_outputs] -> slr_VHAL_TargetType_enum/1
  slr_VHAL_TargetType_enum/1 -> TargetType/1  "<VHAL_TargetType_enum>"
  True_VHAL_TargetType_enum/1 -> TargetType/2
  [inp_CanValid_bus] -> slr1_11/1
  slr1_11/1 -> TargetType/3  "<VINP_CANMsgValidFCM4_flg>"
  TargetType/1 -> VINP_TargetType_enum/1  "VINP_TargetType_enum"
  TargetType/2 -> Terminator_11/1
  [BHAL_outputs] -> slr_VHAL_TimeGapLevel_enum/1
  slr_VHAL_TimeGapLevel_enum/1 -> TimeGapLevel/1  "<VHAL_TimeGapLevel_enum>"
  True_VHAL_TimeGapLevel_enum/1 -> TimeGapLevel/2
  [inp_CanValid_bus] -> slr1_12/1
  slr1_12/1 -> TimeGapLevel/3  "<VINP_CANMsgValidFCM4_flg>"
  TimeGapLevel/1 -> VINP_TimeGapLevel_enum/1  "VINP_TimeGapLevel_enum"
  TimeGapLevel/2 -> Terminator_12/1

== system inp/INP/CAN1/SignalCheck/SRR1 ==
  BHAL_outputs : Inport
  inp_CanValid_bus : Inport  Port=2
  SRRBSDWarnL : FVT_lib/inp/can_signal_template  SystemSampleTime=-1  VariantActivationTime=update diagram  Latency=0  AutoFrameSizeCalculation=off
      link override defval: Value=KINP_SRRBSDWarnL_enum_defval
      link override fftdec: Value=KINP_SRRBSDWarnL_enum_fftdec
      link override fftinc: Value=KINP_SRRBSDWarnL_enum_fftinc
      link override fftlim: Value=KINP_SRRBSDWarnL_enum_fftlim
      link override invalid: Value=KINP_SRRBSDWarnL_enum_invalid
      link override ovrdflg: Value=KINP_SRRBSDWarnL_enum_ovrdflg
      link override ovrdval: Value=KINP_SRRBSDWarnL_enum_ovrdval
      link override setvalid: Value=KINP_SRRBSDWarnL_enum_setvalid
      link override srvcflg: Value=KINP_SRRBSDWarnL_enum_srvcflg
      link override srvcval: Value=KINP_SRRBSDWarnL_enum_srvcval
  SRRBSDWarnR : FVT_lib/inp/can_signal_template  SystemSampleTime=-1  VariantActivationTime=update diagram  Latency=0  AutoFrameSizeCalculation=off
      link override defval: Value=KINP_SRRBSDWarnR_enum_defval
      link override fftdec: Value=KINP_SRRBSDWarnR_enum_fftdec
      link override fftinc: Value=KINP_SRRBSDWarnR_enum_fftinc
      link override fftlim: Value=KINP_SRRBSDWarnR_enum_fftlim
      link override invalid: Value=KINP_SRRBSDWarnR_enum_invalid
      link override ovrdflg: Value=KINP_SRRBSDWarnR_enum_ovrdflg
      link override ovrdval: Value=KINP_SRRBSDWarnR_enum_ovrdval
      link override setvalid: Value=KINP_SRRBSDWarnR_enum_setvalid
      link override srvcflg: Value=KINP_SRRBSDWarnR_enum_srvcflg
      link override srvcval: Value=KINP_SRRBSDWarnR_enum_srvcval
  SRRODAWarnL : FVT_lib/inp/can_signal_template  SystemSampleTime=-1  VariantActivationTime=update diagram  Latency=0  AutoFrameSizeCalculation=off
      link override defval: Value=KINP_SRRODAWarnL_enum_defval
      link override fftdec: Value=KINP_SRRODAWarnL_enum_fftdec
      link override fftinc: Value=KINP_SRRODAWarnL_enum_fftinc
      link override fftlim: Value=KINP_SRRODAWarnL_enum_fftlim
      link override invalid: Value=KINP_SRRODAWarnL_enum_invalid
      link override ovrdflg: Value=KINP_SRRODAWarnL_enum_ovrdflg
      link override ovrdval: Value=KINP_SRRODAWarnL_enum_ovrdval
      link override setvalid: Value=KINP_SRRODAWarnL_enum_setvalid
      link override srvcflg: Value=KINP_SRRODAWarnL_enum_srvcflg
      link override srvcval: Value=KINP_SRRODAWarnL_enum_srvcval
  SRRODAWarnR : FVT_lib/inp/can_signal_template  SystemSampleTime=-1  VariantActivationTime=update diagram  Latency=0  AutoFrameSizeCalculation=off
      link override defval: Value=KINP_SRRODAWarnR_enum_defval
      link override fftdec: Value=KINP_SRRODAWarnR_enum_fftdec
      link override fftinc: Value=KINP_SRRODAWarnR_enum_fftinc
      link override fftlim: Value=KINP_SRRODAWarnR_enum_fftlim
      link override invalid: Value=KINP_SRRODAWarnR_enum_invalid
      link override ovrdflg: Value=KINP_SRRODAWarnR_enum_ovrdflg
      link override ovrdval: Value=KINP_SRRODAWarnR_enum_ovrdval
      link override setvalid: Value=KINP_SRRODAWarnR_enum_setvalid
      link override srvcflg: Value=KINP_SRRODAWarnR_enum_srvcflg
      link override srvcval: Value=KINP_SRRODAWarnR_enum_srvcval
  Terminator_{1..4} (4 alike) : Terminator
  True_VHAL_SRRBSDWarnL_enum : Constant  Value=TRUE  OutDataTypeStr=boolean
  True_VHAL_SRRBSDWarnR_enum : Constant  Value=TRUE  OutDataTypeStr=boolean
  True_VHAL_SRRODAWarnL_enum : Constant  Value=TRUE  OutDataTypeStr=boolean
  True_VHAL_SRRODAWarnR_enum : Constant  Value=TRUE  OutDataTypeStr=boolean
  slr1_{1..4} (4 alike) : BusSelector  OutputSignals=VINP_CANMsgValidSRR1_flg
  slr_VHAL_SRRBSDWarnL_enum : BusSelector  OutputSignals=VHAL_SRRBSDWarnL_enum
  slr_VHAL_SRRBSDWarnR_enum : BusSelector  OutputSignals=VHAL_SRRBSDWarnR_enum
  slr_VHAL_SRRODAWarnL_enum : BusSelector  OutputSignals=VHAL_SRRODAWarnL_enum
  slr_VHAL_SRRODAWarnR_enum : BusSelector  OutputSignals=VHAL_SRRODAWarnR_enum
  VINP_SRRBSDWarnL_enum : Outport
  VINP_SRRBSDWarnR_enum : Outport  Port=2
  VINP_SRRODAWarnL_enum : Outport  Port=3
  VINP_SRRODAWarnR_enum : Outport  Port=4
  wires:
  BHAL_outputs/1 -> [BHAL_outputs]
  inp_CanValid_bus/1 -> [inp_CanValid_bus]
  [BHAL_outputs] -> slr_VHAL_SRRBSDWarnL_enum/1
  slr_VHAL_SRRBSDWarnL_enum/1 -> SRRBSDWarnL/1  "<VHAL_SRRBSDWarnL_enum>"
  True_VHAL_SRRBSDWarnL_enum/1 -> SRRBSDWarnL/2
  [inp_CanValid_bus] -> slr1_1/1
  slr1_1/1 -> SRRBSDWarnL/3  "<VINP_CANMsgValidSRR1_flg>"
  SRRBSDWarnL/1 -> VINP_SRRBSDWarnL_enum/1  "VINP_SRRBSDWarnL_enum"
  SRRBSDWarnL/2 -> Terminator_1/1
  [BHAL_outputs] -> slr_VHAL_SRRBSDWarnR_enum/1
  slr_VHAL_SRRBSDWarnR_enum/1 -> SRRBSDWarnR/1  "<VHAL_SRRBSDWarnR_enum>"
  True_VHAL_SRRBSDWarnR_enum/1 -> SRRBSDWarnR/2
  [inp_CanValid_bus] -> slr1_2/1
  slr1_2/1 -> SRRBSDWarnR/3  "<VINP_CANMsgValidSRR1_flg>"
  SRRBSDWarnR/1 -> VINP_SRRBSDWarnR_enum/1  "VINP_SRRBSDWarnR_enum"
  SRRBSDWarnR/2 -> Terminator_2/1
  [BHAL_outputs] -> slr_VHAL_SRRODAWarnL_enum/1
  slr_VHAL_SRRODAWarnL_enum/1 -> SRRODAWarnL/1  "<VHAL_SRRODAWarnL_enum>"
  True_VHAL_SRRODAWarnL_enum/1 -> SRRODAWarnL/2
  [inp_CanValid_bus] -> slr1_3/1
  slr1_3/1 -> SRRODAWarnL/3  "<VINP_CANMsgValidSRR1_flg>"
  SRRODAWarnL/1 -> VINP_SRRODAWarnL_enum/1  "VINP_SRRODAWarnL_enum"
  SRRODAWarnL/2 -> Terminator_3/1
  [BHAL_outputs] -> slr_VHAL_SRRODAWarnR_enum/1
  slr_VHAL_SRRODAWarnR_enum/1 -> SRRODAWarnR/1  "<VHAL_SRRODAWarnR_enum>"
  True_VHAL_SRRODAWarnR_enum/1 -> SRRODAWarnR/2
  [inp_CanValid_bus] -> slr1_4/1
  slr1_4/1 -> SRRODAWarnR/3  "<VINP_CANMsgValidSRR1_flg>"
  SRRODAWarnR/1 -> VINP_SRRODAWarnR_enum/1  "VINP_SRRODAWarnR_enum"
  SRRODAWarnR/2 -> Terminator_4/1
